simulink model "Traffic_Light_System"  (R2020b)
settings: Solver=FixedStepAuto  StartTime=0.0  StopTime=150  FixedStep=0.1  RelTol=1e-3
undefined symbols (not defined in the file): DiscIntNeverNeededParam
libraries: simulink x1
settings Model: Creator=shubham sharma  LastModifiedBy=shubham sharma

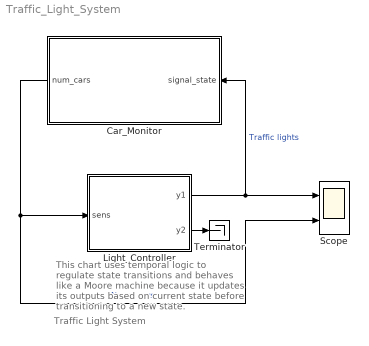
== system Traffic_Light_System ==
  note: Traffic Light System
  note: This chart uses temporal logic to regulate state transitions and
      | behaves like a Moore machine because it updates its outputs
      | based on current state before transitioning to a new state.
  Car_Monitor : Subsystem
  Light_Controller : Stateflow chart  TreatAsAtomicUnit=on
  Scope : Scope  NumInputPorts=2
  Terminator : Terminator
  wires:
  Car_Monitor/1(num_cars) -> Light_Controller/1(sens), Scope/2  "No. of cars"
  Light_Controller/2(y2) -> Terminator/1
  Light_Controller/1(y1) -> Scope/1, Car_Monitor/1(signal_state)  "Traffic lights"

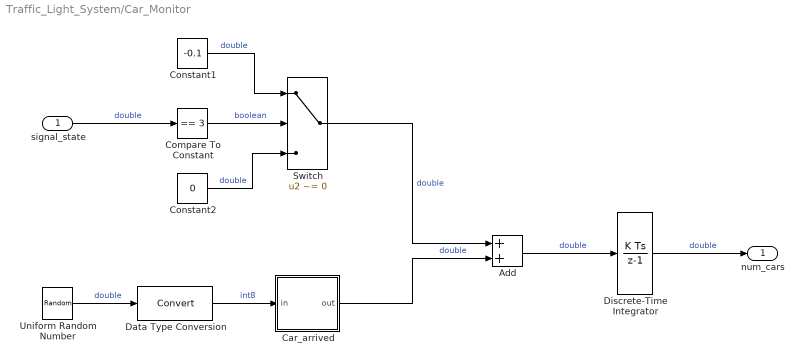
== system Traffic_Light_System/Car_Monitor ==
  signal_state : Inport
  Add : Sum
  Car_arrived : Stateflow chart  TreatAsAtomicUnit=on
  Compare To Constant : simulink/Logic and Bit Operations/Compare To Constant  relop===  const=3  OutDataTypeStr=boolean  ZeroCross=off
  Constant1 : Constant  Value=-0.1
  Constant2 : Constant  Value=0
  Data Type Conversion : DataTypeConversion
  Discrete-Time Integrator : DiscreteIntegrator  SampleTime=-1  LimitOutput=on  LowerSaturationLimit=0  ICPrevOutput=DiscIntNeverNeededParam  ICPrevScaledInput=DiscIntNeverNeededParam
  Switch : Switch  Criteria=u2 ~= 0
  Uniform Random Number : UniformRandomNumber  Minimum=0  Maximum=100  Seed=177836  SampleTime=0
  num_cars : Outport  VectorParamsAs1DForOutWhenUnconnected=off
  wires:
  Constant1/1 -> Switch/1  "double"
  Constant2/1 -> Switch/3  "double"
  Discrete-Time Integrator/1 -> num_cars/1  "double"
  signal_state/1 -> Compare To Constant/1  "double"
  Compare To Constant/1 -> Switch/2  "boolean"
  Switch/1 -> Add/1  "double"
  Add/1 -> Discrete-Time Integrator/1  "double"
  Car_arrived/1(out) -> Add/2  "double"
  Data Type Conversion/1 -> Car_arrived/1(in)  "int8"
  Uniform Random Number/1 -> Data Type Conversion/1  "double"

== stateflow chart Traffic_Light_System/Light_Controller ==
  settings: stateMachineType=MOORE_MACHINE  executeAtInitialization=1  initializeOutput=1
  note: Traffic light has been green for North-South,
      | red for East-West for 10 clock ticks.
  note: Traffic light has been red for North-South,
      | yellow for East-West for 3 clock ticks.
  state GoToStop
    y1 = YELLOW;
    y2 = RED;
  state Go
    y1 = GREEN;
    y2 = RED;
  note: If sensor indicates cars are waiting ([sens] is true) in the
      | North-South direction, active state becomes StopToGo.
  state Stop
    y1 = RED;
    y2 = GREEN;
  state StopForTraffic
    y1 = RED;
    y2 = GREEN;
  state StopToGo
    y1 = RED;
    y2 = YELLOW;
  note: Traffic light is red for North-South,
      | green for East-West.
  note: Traffic light has been red for North-South,
      | green for East-West for at least 20 clock ticks.
  note: Traffic light must reverse traffic flow in
      | response to sensor.
  Go -> GoToStop : after(10,tick)
  GoToStop -> Stop : after (3,tick)
  StopToGo -> Go : after(3,tick)
  StopForTraffic -> StopToGo : [sens]
  (default) -> Stop
  Stop -> StopForTraffic : after(20,tick)
  data: sens input double; y1 output double; RED constant uint8 =1; YELLOW constant double =2; GREEN constant double =3; y2 output double

== stateflow chart Traffic_Light_System/Car_Monitor/Car_arrived ==
  (default) -> (junction 2) : {out = in > 98;}
  data: in input int8; out output double
